simulink model "RSC_1_2"  (R2019a)
settings: Solver=FixedStepAuto  StartTime=0.0  StopTime=T  RelTol=1e-3
settings Model: Creator=vanka  LastModifiedBy=vanka
settings DataIOCC: ReturnWorkspaceOutputs=off
settings DebuggingCC: PregeneratedLibrarySubsystemCodeDiagnostic=none  ArithmeticOperatorsInVariantConditions=warning
settings SFSimCC: SimUseLocalCustomCode=off
settings RTWCC: RTWUseLocalCustomCode=off

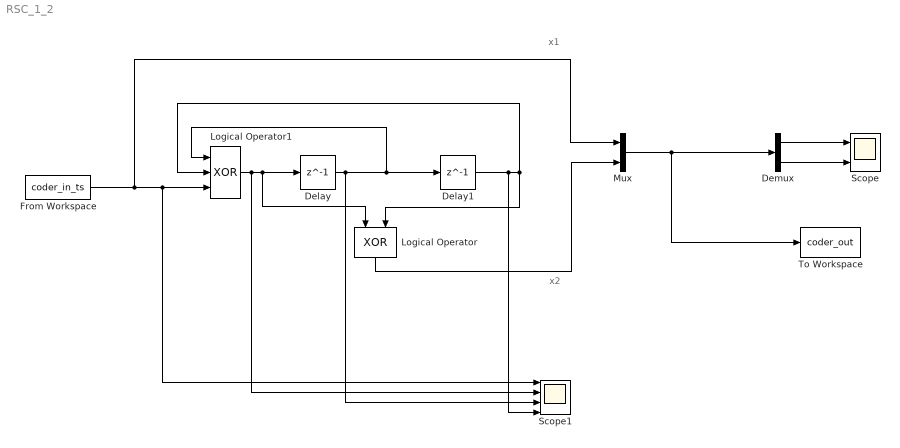
== system RSC_1_2 ==
  note: x2
  note: x1
  Delay : Delay  DelayLength=1  SampleTime=1
  Delay1 : Delay  DelayLength=1  SampleTime=1
  Demux : Demux  Outputs=2
  From Workspace : FromWorkspace  VariableName=coder_in_ts  OutDataTypeStr=boolean  SampleTime=1
  Logical Operator : Logic  Operator=XOR  IconShape=distinctive  AllPortsSameDT=off  OutDataTypeStr=boolean
  Logical Operator1 : Logic  Operator=XOR  Inputs=3  IconShape=distinctive  AllPortsSameDT=off  OutDataTypeStr=boolean
  Mux : Mux  Inputs=2
  Scope : Scope  NumInputPorts=2
  Scope1 : Scope  NumInputPorts=4
  To Workspace : ToWorkspace  VariableName=coder_out  SaveFormat=Timeseries  SampleTime=1
  wires:
  Logical Operator1/1 -> Scope1/2, Logical Operator/1, Delay/1
  Delay/1 -> Logical Operator1/1, Delay1/1, Scope1/3
  Delay1/1 -> Scope1/4, Logical Operator1/2, Logical Operator/2
  From Workspace/1 -> Mux/1, Scope1/1, Logical Operator1/3
  Logical Operator/1 -> Mux/2
  Mux/1 -> To Workspace/1, Demux/1
  Demux/1 -> Scope/1
  Demux/2 -> Scope/2
